simulink model "lab009_sim_1"  (R2017b)
settings: Solver=FixedStepAuto  StartTime=0.0  StopTime=30.0  FixedStep=1e-3  RelTol=1e-3
values from neighbouring files (symbols this model uses):
  c = 0.3    [lab008_1.m]    (also in lab009_1.m = [0.1 0.1 0.15])
  k = 1000    [lab008_1.m]    (also in lab009_1.m = [1000 1500 2000])
  m = 2    [lab008_1.m]    (also in lab009_1.m = [0.8 1])
libraries: simulink x1
settings Model: Creator=kamzab95  LastModifiedBy=kamzab95

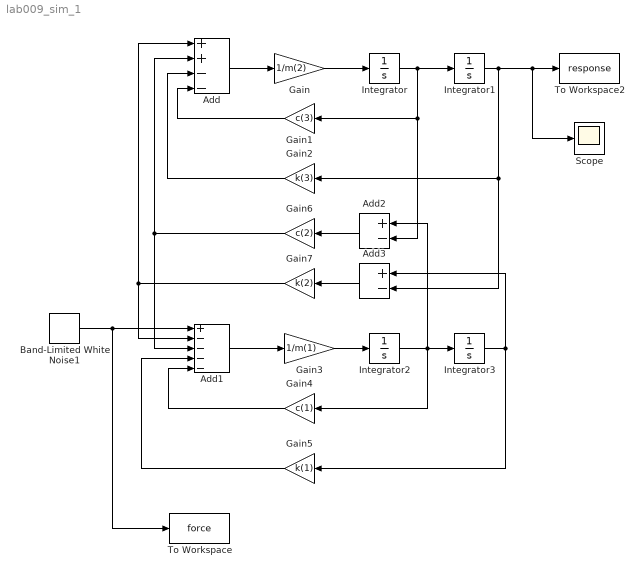
== system lab009_sim_1 ==
  Add : Sum  Inputs=++--
  Add1 : Sum  Inputs=+----
  Add2 : Sum  Inputs=+-
  Add3 : Sum  Inputs=+-
  Band-Limited White Noise1 : simulink/Sources/Band-Limited White Noise  Cov=[0.1]  Ts=1e-3  seed=[23341]
  Gain : Gain  Gain=1/m(2)
  Gain1 : Gain  Gain=c(3)
  Gain2 : Gain  Gain=k(3)
  Gain3 : Gain  Gain=1/m(1)
  Gain4 : Gain  Gain=c(1)
  Gain5 : Gain  Gain=k(1)
  Gain6 : Gain  Gain=c(2)
  Gain7 : Gain  Gain=k(2)
  Integrator{,1..3} (4 alike) : Integrator
  Scope : Scope
  To Workspace : ToWorkspace  VariableName=force  SaveFormat=Timeseries  SampleTime=-1
  To Workspace2 : ToWorkspace  VariableName=response  SaveFormat=Timeseries  SampleTime=-1
  wires:
  Gain/1 -> Integrator/1
  Add/1 -> Gain/1
  Integrator/1 -> Add2/2, Gain1/1, Integrator1/1
  Gain5/1 -> Add1/4
  Gain3/1 -> Integrator2/1
  Integrator3/1 -> Add3/1, Gain5/1
  Integrator2/1 -> Add2/1, Gain4/1, Integrator3/1
  Gain4/1 -> Add1/5
  Gain2/1 -> Add/3
  Gain1/1 -> Add/4
  Integrator1/1 -> Scope/1, To Workspace2/1, Add3/2, Gain2/1
  Add3/1 -> Gain7/1
  Add2/1 -> Gain6/1
  Gain6/1 -> Add/2, Add1/3
  Gain7/1 -> Add/1, Add1/2
  Band-Limited White Noise1/1 -> To Workspace/1, Add1/1
  Add1/1 -> Gain3/1
